simulink model "TV"  (R2025b)
settings: Solver=ode4  StartTime=0.0  StopTime=10.0  FixedStep=0.0005  RelTol=1e-3
undefined symbols (not defined in the file): tv
Description:
  | Adapted De Novellis et al. (IEEE TVT 2014) feedforward + PID TV controller.
settings Model: Creator=jaiden  LastModifiedBy=r3anjum

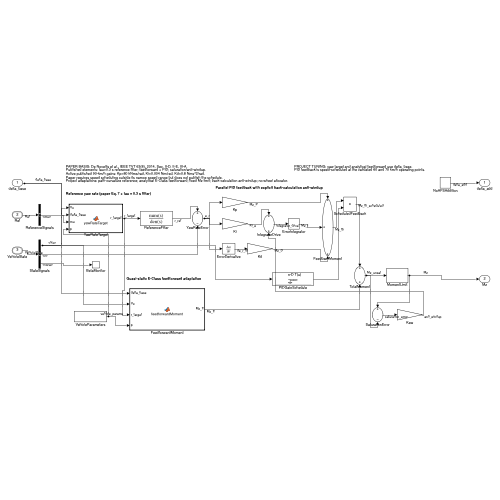
[thumbnail: Simulink's stored preview of the top-level diagram]
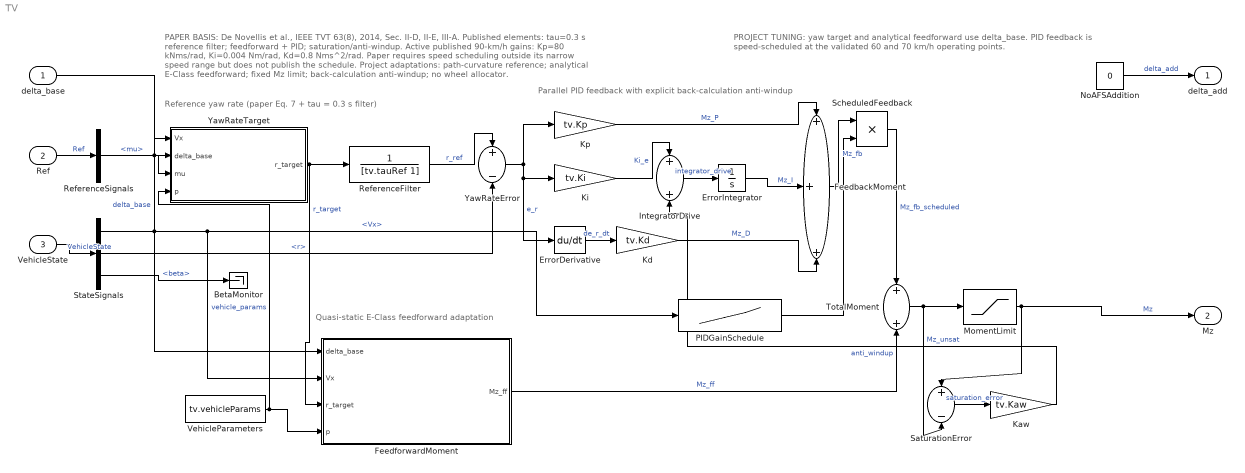
== system TV ==
  note: PAPER BASIS: De Novellis et al., IEEE TVT 63(8), 2014, Sec. II-D, II-E, III-A.
      | Published elements: tau=0.3 s reference filter; feedforward + PID; saturation/anti-windup.
      | Active published 90-km/h gains: Kp=80 kNms/rad, Ki=0.004 Nm/rad, Kd=0.8 Nms^2/rad.
      | Paper requires speed scheduling outside its narrow speed range but does not publish the schedule.
      | Project adaptations: path-curvature reference; analytical E-Class feedforward; fixed Mz limit; back-calculation anti-windup; no wheel allocator.
  note: Reference yaw rate (paper Eq. 7 + tau = 0.3 s filter)
  note: Parallel PID feedback with explicit back-calculation anti-windup
  note: Quasi-static E-Class feedforward adaptation
  note: PROJECT TUNING: yaw target and analytical feedforward use delta_base.
      | PID feedback is speed-scheduled at the validated 60 and 70 km/h operating points.
  delta_base : Inport
  Ref : Inport  Port=2  OutDataTypeStr=Bus: ReferenceBus
  VehicleState : Inport  Port=3  OutDataTypeStr=Bus: VehicleStateBus
  BetaMonitor : Terminator
  ErrorDerivative : Derivative
  ErrorIntegrator : Integrator
  FeedbackMoment : Sum  Inputs=+++
  FeedforwardMoment : MATLAB Function  TreatAsAtomicUnit=on
  IntegratorDrive : Sum  Description=Integral drive = Ki*e_r + Kaw*(Mz-Mz_unsat). The paper states
  Kaw : Gain  Description=Project-specific back-calculation gain. The paper confirms  Gain=tv.Kaw
  Kd : Gain  Gain=tv.Kd
  Ki : Gain  Gain=tv.Ki
  Kp : Gain  Gain=tv.Kp
  MomentLimit : Saturate  Description=Fixed bicycle-model yaw-moment authority; replace with plant-specific  UpperLimit=tv.MzMax  LowerLimit=-tv.MzMax  ZeroCross=off
  NoAFSAddition : Constant  Value=0
  PIDGainSchedule : Lookup_n-D  NumberOfTableDimensions=1  BreakpointsForDimension1=tv.tuned.speedBreakpoints  Table=tv.tuned.gainScales  ExtrapMethod=Clip  InternalRulePriority=Speed  RndMeth=Simplest
  ReferenceFilter : TransferFcn  Description=Paper Sec. II-D: first-order reference-yaw-rate factor, tau = 0.3 s.  Numerator=1  Denominator=[tv.tauRef 1]
  ReferenceSignals : BusSelector  OutputSignals=mu
  SaturationError : Sum  Inputs=+-
  ScheduledFeedback : Product  Inputs=**
  StateSignals : BusSelector  OutputSignals=Vx,r,beta
  TotalMoment : Sum
  VehicleParameters : Constant  Description=[m, a, b, Caf, Car] for analytical E-Class feedforward.  Value=tv.vehicleParams
  YawRateError : Sum  Description=e_r = r_ref - r matches negative feedback in paper Eq. (5) and  Inputs=+-
  YawRateTarget : MATLAB Function  TreatAsAtomicUnit=on
  delta_add : Outport
  Mz : Outport  Port=2
  wires:
  NoAFSAddition/1 -> delta_add/1  "delta_add"
  Ref/1 -> ReferenceSignals/1  "Ref"
  VehicleState/1 -> StateSignals/1  "VehicleState"
  StateSignals/3 -> BetaMonitor/1  "<beta>"
  StateSignals/1 -> FeedforwardMoment/2(Vx), PIDGainSchedule/1, YawRateTarget/1(Vx)  "<Vx>"
  YawRateTarget/1(r_target) -> ReferenceFilter/1, FeedforwardMoment/3(r_target)  "r_target"
  ReferenceFilter/1 -> YawRateError/1  "r_ref"
  StateSignals/2 -> YawRateError/2  "<r>"
  YawRateError/1 -> Ki/1, ErrorDerivative/1, Kp/1  "e_r"
  Ki/1 -> IntegratorDrive/1  "Ki_e"
  IntegratorDrive/1 -> ErrorIntegrator/1  "integrator_drive"
  ErrorDerivative/1 -> Kd/1  "de_r_dt"
  Kp/1 -> FeedbackMoment/1  "Mz_P"
  ErrorIntegrator/1 -> FeedbackMoment/2  "Mz_I"
  Kd/1 -> FeedbackMoment/3  "Mz_D"
  VehicleParameters/1 -> FeedforwardMoment/4(p), YawRateTarget/4(p)  "vehicle_params"
  FeedforwardMoment/1(Mz_ff) -> TotalMoment/2  "Mz_ff"
  TotalMoment/1 -> MomentLimit/1, SaturationError/2  "Mz_unsat"
  MomentLimit/1 -> Mz/1, SaturationError/1  "Mz"
  SaturationError/1 -> Kaw/1  "saturation_error"
  Kaw/1 -> IntegratorDrive/2  "anti_windup"
  ReferenceSignals/1 -> YawRateTarget/3(mu)  "<mu>"
  delta_base/1 -> YawRateTarget/2(delta_base), FeedforwardMoment/1(delta_base)  "delta_base"
  FeedbackMoment/1 -> ScheduledFeedback/1  "Mz_fb"
  PIDGainSchedule/1 -> ScheduledFeedback/2
  ScheduledFeedback/1 -> TotalMoment/1  "Mz_fb_scheduled"

== matlab function TV/FeedforwardMoment ==
  data: delta_base input; Mz_ff output; Vx input; r_target input; p input
function Mz_ff = feedforwardMoment(delta_base, Vx, r_target, p)
%FEEDFORWARDMOMENT Steering-coordinated steady-state yaw moment.
% The same steering command and target are used by feedforward and
% feedback. For the nominal bicycle model this produces approximately
% zero steady moment, leaving TV to correct transient/model mismatch.
m = p(1); a = p(2); b = p(3); Caf = p(4); Car = p(5);
if abs(Vx) < 0.1
    Mz_ff = 0;
    return;
end
Vy_ss = (Caf*Vx*delta_base + (b*Car-a*Caf)*r_target ...
         - m*Vx^2*r_target)/(Caf+Car);
alpha_f = delta_base - (Vy_ss+a*r_target)/Vx;
alpha_r = -(Vy_ss-b*r_target)/Vx;
Fyf_ss = Caf*alpha_f;
Fyr_ss = Car*alpha_r;
Mz_ff = -(a*Fyf_ss-b*Fyr_ss);
end

== matlab function TV/YawRateTarget ==
  data: Vx input; r_target output; delta_base input; mu input; p input
function r_target = yawRateTarget(Vx, delta_base, mu, p)
%YAWRATETARGET Steering-coordinated nominal E-Class response.
% TV regulates the response expected from the steering command that is
% actually sent to the plant. This prevents the TV loop from acting as
% a second path controller with an independent curvature-only target.
m = p(1); a = p(2); b = p(3); Caf = p(4); Car = p(5);
g = 9.81;
L = a + b;
Vx_safe = max(abs(Vx), 0.1);

% Linear-bicycle understeer coefficient and nominal yaw response.
Kus = (m/L)*(b/Caf - a/Car);
denominator = max(L + Kus*Vx^2, 0.1);
r_steer = Vx*delta_base/denominator;

% Friction-limited yaw target.
r_limit = mu*g/Vx_safe;
r_target = min(max(r_steer, -r_limit), r_limit);
end
